simulink model "untitled"  (R2021b)
settings: Solver=VariableStepAuto  StartTime=0.0  StopTime=6.0  RelTol=1e-3
settings Model: Creator=Mahban  LastModifiedBy=Mahban

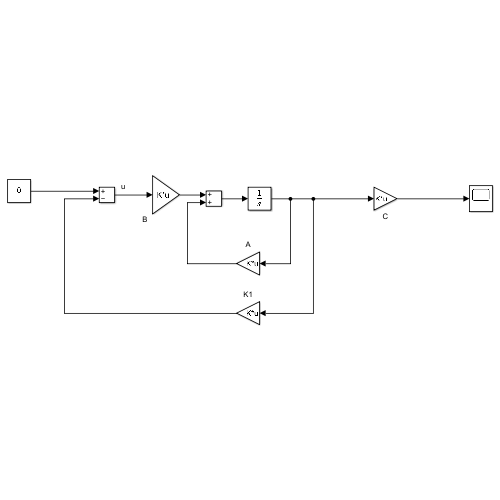
[thumbnail: Simulink's stored preview of the top-level diagram]
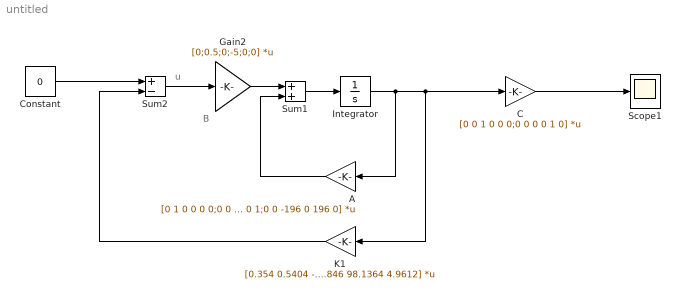
== system untitled ==
  note: u
  note: B
  A : Gain  Gain=[0 1 0 0 0 0;0 0 -0.98 0 0 0;0 0 0 1 0 0;0 0 205.8 0 -98 0;0 0 0 0 0 1;0 0 -196 0 196 0]  Multiplication=Matrix(K*u)
  C : Gain  Gain=[0 0 1 0 0 0;0 0 0 0 1 0]  Multiplication=Matrix(K*u)
  Constant : Constant  Value=0
  Gain2 : Gain  Gain=[0;0.5;0;-5;0;0]  Multiplication=Matrix(K*u)
  Integrator : Integrator  InitialCondition=ones(6,1)
  K1 : Gain  Gain=[0.354 0.5404 -116.4246 -3.846 98.1364 4.9612]  Multiplication=Matrix(K*u)
  Scope1 : Scope
  Sum1 : Sum
  Sum2 : Sum  Inputs=+-
  wires:
  Constant/1 -> Sum2/1
  A/1 -> Sum1/2
  Integrator/1 -> A/1, C/1, K1/1
  Sum2/1 -> Gain2/1
  Sum1/1 -> Integrator/1
  K1/1 -> Sum2/2
  Gain2/1 -> Sum1/1
  C/1 -> Scope1/1
